simulink library "uavsimBlockset_RotationVector2Quaternion"  (Simulink 8.0)
settings: Solver=ode45  StartTime=0.0  StopTime=10.0  RelTol=1e-3
libraries: uavsimblockset x2, aerolibutil x1
settings Model: Creator=mstolle  LastModifiedBy=j.bolting

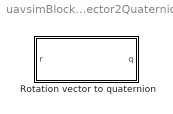
== system uavsimBlockset_RotationVector2Quaternion ==
  Rotation vector to quaternion : Subsystem

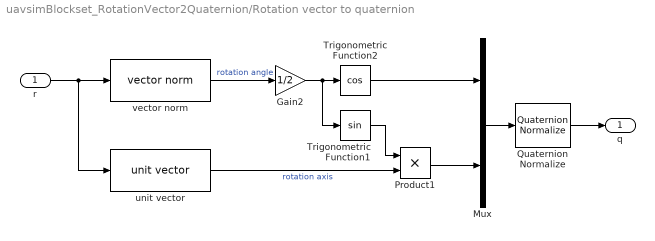
== system uavsimBlockset_RotationVector2Quaternion/Rotation vector to quaternion ==
  r : Inport
  Gain2 : Gain  Gain=1/2
  Mux : Mux  Inputs=2
  Product1 : Product  RndMeth=Zero
  Quaternion Normalize : aerolibutil/Quaternion Normalize
  Trigonometric Function1 : Trigonometry
  Trigonometric Function2 : Trigonometry  Operator=cos
  unit vector : uavsimblockset/unit vector
  vector norm : uavsimblockset/vector norm
  q : Outport
  wires:
  Mux/1 -> Quaternion Normalize/1
  r/1 -> unit vector/1, vector norm/1
  vector norm/1 -> Gain2/1  "rotation angle"
  Gain2/1 -> Trigonometric Function1/1, Trigonometric Function2/1
  Trigonometric Function2/1 -> Mux/1
  unit vector/1 -> Product1/2  "rotation axis"
  Trigonometric Function1/1 -> Product1/1
  Product1/1 -> Mux/2
  Quaternion Normalize/1 -> q/1
